simulink model "pd_nf_pi_dvco"  (R2024b)
settings: configuration reference "CONFI" (kept outside this file)
libraries: slpidlib x1
settings Model: DataDictionary=dic_pfc3ph.sldd  Creator=ASUSTUF  LastModifiedBy=Angel
settings ConfigSetRef: SourceName=CONFI

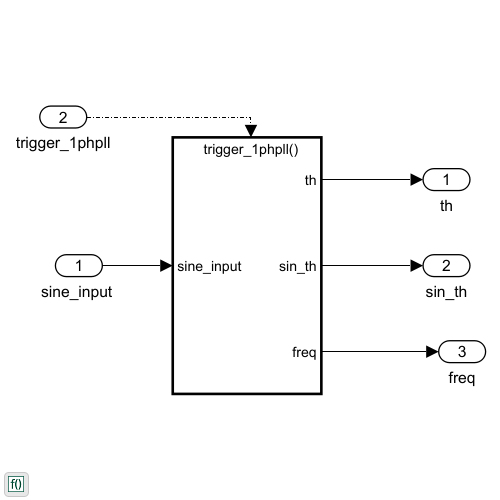
[thumbnail: Simulink's stored preview of the top-level diagram]
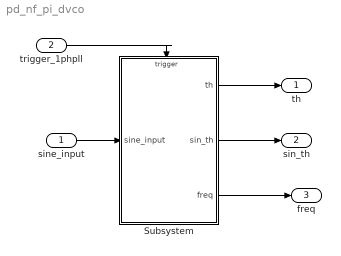
== system pd_nf_pi_dvco ==
  "sine_input " : Inport
  trigger_1phpll : Inport  Port=2  OutputFunctionCall=on
  Subsystem : Subsystem
  th : Outport
  sin_th : Outport  Port=2
  freq : Outport  Port=3
  wires:
  "sine_input "/1 -> Subsystem/1("sine_input ")
  Subsystem/1(th) -> th/1
  Subsystem/2(sin_th) -> sin_th/1
  Subsystem/3(freq) -> freq/1
  trigger_1phpll/1 -> Subsystem/Trigger

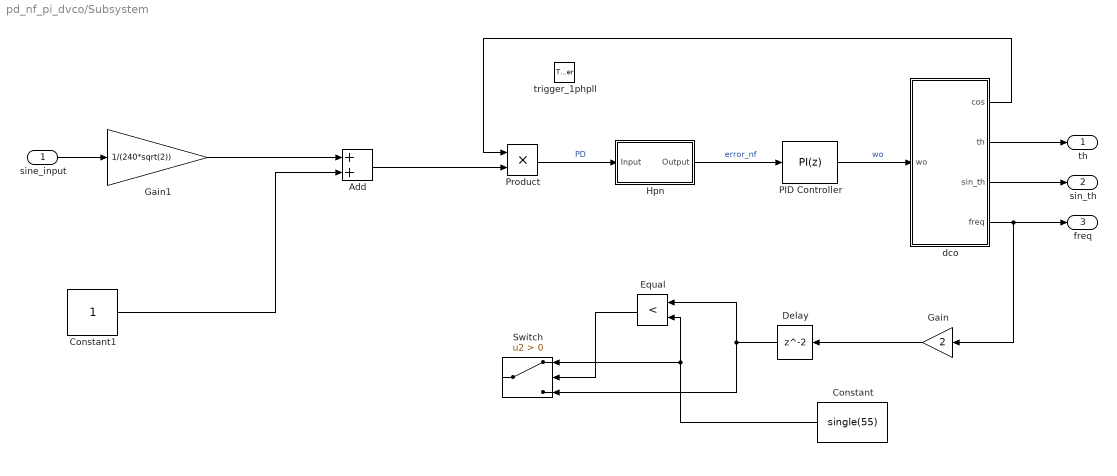
== system pd_nf_pi_dvco/Subsystem ==
  "sine_input " : Inport
  trigger_1phpll : TriggerPort  TriggerType=function-call  VariantControl=(inherit)  PortDimensions=1
  Add : Sum
  Constant : Constant  Value=single(55)  OutDataTypeStr=single  SampleTime=-1
  Constant1 : Constant  OutDataTypeStr=single  SampleTime=-1
  Delay : Delay  InitialCondition=single(2*55)
  Equal : RelationalOperator  Operator=<  OutDataTypeStr=boolean  RndMeth=Simplest  InputSameDT=off
  Gain : Gain  Gain=2  OutDataTypeStr=single
  Gain1 : Gain  Gain=1/(240*sqrt(2))  OutDataTypeStr=single
  Hpn : Subsystem  Tag=FilterWizardSubSystem
      settings: ErrorFcn=dspFilterRealizedInBasicElemsAlgLoopErrFcnCallback
  PID Controller : slpidlib/PID Controller  Controller=PI  Form=Parallel  TimeDomain=Discrete-time  UseExternalTs=on  SampleTime=-1  IntegratorMethod=Forward Euler  FilterMethod=Forward Euler  ControllerParametersSource=internal  P=1  I=.1  UseKiTs=on  D=60  UseExternalDerivativeSource=off  N=5  UseFilter=on  TunerSelectOption=Transfer Function Based (PID Tuner App)  InitialConditionSource=internal  InitialConditionForIntegrator=0  InitialConditionForFilter=0  DifferentiatorICPrevScaledInput=0  ExternalReset=none  TrackingMode=off  Kt=1  LimitOutput=off  SatLimitsSource=internal  UpperSaturationLimit=inf  LowerSaturationLimit=-inf  LinearizeAsGain=on  AntiWindupMode=none  Kb=1  LimitIntegrator=off  UpperIntegratorSaturationLimit=inf  LowerIntegratorSaturationLimit=-inf  PGainOutDataTypeStr=single  PProdOutDataTypeStr=single  POutMin=[]  POutMax=[]  IGainOutDataTypeStr=single  IProdOutDataTypeStr=single  IOutMin=[]  IOutMax=[]  DOutMin=[]  DOutMax=[]  NOutMin=[]  NOutMax=[]  SumOutDataTypeStr=single  SumOutMin=[]  SumOutMax=[]  SaturationOutMin=[]  SaturationOutMax=[]  PParamMin=[]  PParamMax=[]  IParamMin=[]  IParamMax=[]  DParamMin=[]  DParamMax=[]  NParamMin=[]  NParamMax=[]  KbParamMin=[]  KbParamMax=[]  KtParamMin=[]  KtParamMax=[]  KbOutMin=[]  KbOutMax=[]  KtOutMin=[]  KtOutMax=[]  IntegratorOutMin=[]  IntegratorOutMax=[]  FilterOutMin=[]  FilterOutMax=[]  SumI1OutMin=[]  SumI1OutMax=[]  SumI2OutMin=[]  SumI2OutMax=[]  SumI3OutMin=[]  SumI3OutMax=[]  SumI4OutMin=[]  SumI4OutMax=[]  SumDOutMin=[]  SumDOutMax=[]  DifferentiatorOutMin=[]  DifferentiatorOutMax=[]  FilterDiffOutCoefMin=[]  FilterDiffOutCoefMax=[]  ReciprocalOutMin=[]  ReciprocalOutMax=[]  SumDenOutMin=[]  SumDenOutMax=[]  SumNumOutMin=[]  SumNumOutMax=[]  DivideOutMin=[]  DivideOutMax=[]  UdiffTsProdOutMin=[]  UdiffTsProdOutMax=[]  NTsProdOutMin=[]  NTsProdOutMax=[]  UintegralTsProdOutMin=[]  UintegralTsProdOutMax=[]  UngainTsProdOutMin=[]  UngainTsProdOutMax=[]  ClampingZeroOutDataTypeStr=Inherit: Inherit via back propagation  ClampingZeroOutMin=[]  ClampingZeroOutMax=[]  FilterDenConstantOutDataTypeStr=Inherit: Inherit via back propagation  FilterDenConstantOutMin=[]  FilterDenConstantOutMax=[]  PCopyOutDataTypeStr=Inherit: Inherit via back propagation  PCopyOutMin=[]  PCopyOutMax=[]  NCopyOutDataTypeStr=Inherit: Inherit via back propagation  NCopyOutMin=[]  NCopyOutMax=[]  IntegratorContinuousStateAttributes=''  IntegratorStateMustResolveToSignalObject=off  IntegratorRTWStateStorageClass=Auto  FilterContinuousStateAttributes=''  FilterStateMustResolveToSignalObject=off  FilterRTWStateStorageClass=Auto  ParallelPVariant=InternalParameters  IdealPVariant=Disabled  IVariant=InternalParameters  DVariant=Disabled  IntegratorVariant=Discrete  SatVariant=Disabled  AWVariant=Passthrough  PCopyVariant=Disabled  TRVariant=Disabled  FdbkBlocksVariant=Forward  IdealPFdbkVariant=Disabled  SatFdbkVariant=Disabled  DerivativeFilterVariant=Disabled  NVariant=Disabled  NCopyVariant=Disabled_SignalSpec  FilterICVariant=Disabled  IntegratorICVariant=InternalICs  ExternalResetVariant=Disabled  TRSumVariant=Passthrough  SumFdbkVariant=Disabled  SumVariant=Sum_PI  TsampFilterVariant=InternalTs  TsampNgainVariant=Passthrough  TsampIntegralVariant=Passthrough  ExternalSaturationOutDataTypeStr=Inherit: Same as second input  DerivativeSourceVariant=Disabled  PreIntVariant=InternalPreInt
  Product : Product  OutDataTypeStr=single
  Switch : Switch  Criteria=u2 > Threshold  SaturateOnIntegerOverflow=off  InputSameDT=off
  dco : Subsystem
  th : Outport
  sin_th : Outport  Port=2
  freq : Outport  Port=3
  wires:
  dco/1(cos) -> Product/1
  Product/1 -> Hpn/1(Input)  "PD"
  Constant1/1 -> Add/2
  PID Controller/1 -> dco/1(wo)  "wo"
  Equal/1 -> Switch/2
  Gain/1 -> Delay/1
  Hpn/1(Output) -> PID Controller/1  "error_nf"
  dco/3(sin_th) -> sin_th/1
  dco/4(freq) -> freq/1, Gain/1
  "sine_input "/1 -> Gain1/1
  dco/2(th) -> th/1
  Constant/1 -> Switch/1, Equal/2
  Add/1 -> Product/2
  Delay/1 -> Switch/3, Equal/1
  Gain1/1 -> Add/1

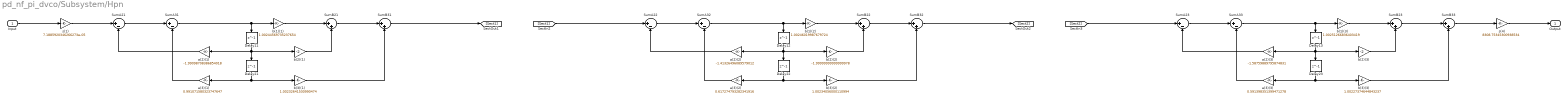
== system pd_nf_pi_dvco/Subsystem/Hpn ==
  Input : Inport
  Delay{11..13,21..23} (6 alike) : Delay  DelayLength=1  InitialCondition=0
  SumA{21..23,31..33} (6 alike) : Sum  Inputs=|+-  RndMeth=Nearest  SaturateOnIntegerOverflow=on  OutDataTypeStr=Inherit: Same as first input
  SumB{21..23,31..33} (6 alike) : Sum  Inputs=|++  RndMeth=Nearest  SaturateOnIntegerOverflow=on  OutDataTypeStr=Inherit: Same as first input
  a(2)(1) : Gain  Gain=-1.99098708386854018  ParamDataTypeStr=single  RndMeth=Nearest  SaturateOnIntegerOverflow=on  OutDataTypeStr=Inherit: Same as input
  a(2)(2) : Gain  Gain=-1.41326496089579012  ParamDataTypeStr=single  RndMeth=Nearest  SaturateOnIntegerOverflow=on  OutDataTypeStr=Inherit: Same as input
  a(2)(3) : Gain  Gain=-1.58759889795874831  ParamDataTypeStr=single  RndMeth=Nearest  SaturateOnIntegerOverflow=on  OutDataTypeStr=Inherit: Same as input
  a(3)(1) : Gain  Gain=0.991071580323747647  ParamDataTypeStr=single  RndMeth=Nearest  SaturateOnIntegerOverflow=on  OutDataTypeStr=Inherit: Same as input
  a(3)(2) : Gain  Gain=0.617274793282341916  ParamDataTypeStr=single  RndMeth=Nearest  SaturateOnIntegerOverflow=on  OutDataTypeStr=Inherit: Same as input
  a(3)(3) : Gain  Gain=0.591398351399471278  ParamDataTypeStr=single  RndMeth=Nearest  SaturateOnIntegerOverflow=on  OutDataTypeStr=Inherit: Same as input
  b(1)(1) : Gain  Gain=1.00244569735237654  ParamDataTypeStr=single  RndMeth=Nearest  SaturateOnIntegerOverflow=on  OutDataTypeStr=Inherit: Same as input
  b(1)(2) : Gain  Gain=1.00246019987679724  ParamDataTypeStr=single  RndMeth=Nearest  SaturateOnIntegerOverflow=on  OutDataTypeStr=Inherit: Same as input
  b(1)(3) : Gain  Gain=1.00251266836403419  ParamDataTypeStr=single  RndMeth=Nearest  SaturateOnIntegerOverflow=on  OutDataTypeStr=Inherit: Same as input
  b(2)(1) : Gain  Gain=-2  ParamDataTypeStr=single  RndMeth=Nearest  SaturateOnIntegerOverflow=on  OutDataTypeStr=Inherit: Same as input
  b(2)(2) : Gain  Gain=-1.99999999999999978  ParamDataTypeStr=single  RndMeth=Nearest  SaturateOnIntegerOverflow=on  OutDataTypeStr=Inherit: Same as input
  b(2)(3) : Gain  Gain=-2  ParamDataTypeStr=single  RndMeth=Nearest  SaturateOnIntegerOverflow=on  OutDataTypeStr=Inherit: Same as input
  b(3)(1) : Gain  Gain=1.00232641530990474  ParamDataTypeStr=single  RndMeth=Nearest  SaturateOnIntegerOverflow=on  OutDataTypeStr=Inherit: Same as input
  b(3)(2) : Gain  Gain=1.00234056000110994  ParamDataTypeStr=single  RndMeth=Nearest  SaturateOnIntegerOverflow=on  OutDataTypeStr=Inherit: Same as input
  b(3)(3) : Gain  Gain=1.00227374644843237  ParamDataTypeStr=single  RndMeth=Nearest  SaturateOnIntegerOverflow=on  OutDataTypeStr=Inherit: Same as input
  s(1) : Gain  Gain=7.1885920346266273e-05  ParamDataTypeStr=single  RndMeth=Nearest  SaturateOnIntegerOverflow=on  OutDataTypeStr=Inherit: Same as input
  s(4) : Gain  Gain=8308.75345300938534  ParamDataTypeStr=single  RndMeth=Nearest  SaturateOnIntegerOverflow=on  OutDataTypeStr=Inherit: Same as input
  Output : Outport
  wires:
  Input/1 -> s(1)/1
  s(1)/1 -> SumA21/1
  SumA21/1 -> SumA31/1
  SumA31/1 -> b(1)(1)/1, Delay11/1
  b(1)(1)/1 -> SumB21/1
  SumB21/1 -> SumB31/1
  SumB31/1 -> [Sect1]
  a(2)(1)/1 -> SumA21/2
  Delay11/1 -> a(2)(1)/1, b(2)(1)/1, Delay21/1
  b(2)(1)/1 -> SumB21/2
  a(3)(1)/1 -> SumA31/2
  Delay21/1 -> a(3)(1)/1, b(3)(1)/1
  b(3)(1)/1 -> SumB31/2
  [Sect1] -> SumA22/1
  SumA22/1 -> SumA32/1
  SumA32/1 -> b(1)(2)/1, Delay12/1
  b(1)(2)/1 -> SumB22/1
  SumB22/1 -> SumB32/1
  SumB32/1 -> [Sect2]
  a(2)(2)/1 -> SumA22/2
  Delay12/1 -> a(2)(2)/1, b(2)(2)/1, Delay22/1
  b(2)(2)/1 -> SumB22/2
  a(3)(2)/1 -> SumA32/2
  Delay22/1 -> a(3)(2)/1, b(3)(2)/1
  b(3)(2)/1 -> SumB32/2
  [Sect2] -> SumA23/1
  SumA23/1 -> SumA33/1
  SumA33/1 -> b(1)(3)/1, Delay13/1
  b(1)(3)/1 -> SumB23/1
  SumB23/1 -> SumB33/1
  SumB33/1 -> s(4)/1
  a(2)(3)/1 -> SumA23/2
  Delay13/1 -> a(2)(3)/1, b(2)(3)/1, Delay23/1
  b(2)(3)/1 -> SumB23/2
  a(3)(3)/1 -> SumA33/2
  Delay23/1 -> a(3)(3)/1, b(3)(3)/1
  b(3)(3)/1 -> SumB33/2
  s(4)/1 -> Output/1

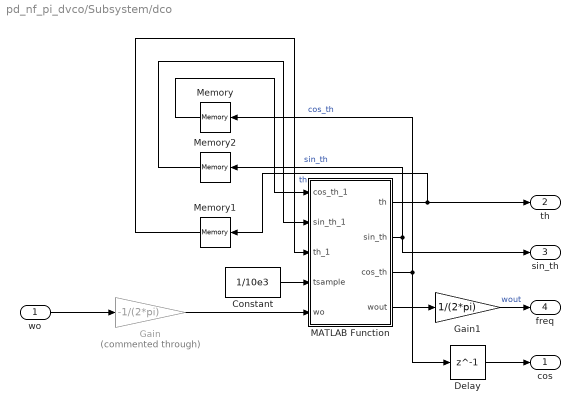
== system pd_nf_pi_dvco/Subsystem/dco ==
  wo : Inport
  Constant : Constant  Value=1/10e3  OutDataTypeStr=single  SampleTime=-1
  Delay : Delay  DelayLength=1  InitialCondition=single(0')
  Gain : Gain  Commented=through  Gain=-1/(2*pi)
  Gain1 : Gain  Gain=1/(2*pi)  OutDataTypeStr=single
  MATLAB Function : MATLAB Function  TreatAsAtomicUnit=on
  Memory : Memory  InitialCondition=.99  InheritSampleTime=on
  Memory1 : Memory  InheritSampleTime=on
  Memory2 : Memory  InheritSampleTime=on
  cos : Outport
  th : Outport  Port=2
  sin_th : Outport  Port=3
  freq : Outport  Port=4
  wires:
  wo/1 -> Gain/1
  Constant/1 -> MATLAB Function/4(tsample)
  Memory1/1 -> MATLAB Function/3(th_1)
  Memory2/1 -> MATLAB Function/2(sin_th_1)
  Memory/1 -> MATLAB Function/1(cos_th_1)
  Delay/1 -> cos/1
  MATLAB Function/1(th) -> Memory1/1, th/1  "th"
  MATLAB Function/2(sin_th) -> sin_th/1, Memory2/1  "sin_th"
  MATLAB Function/3(cos_th) -> Delay/1, Memory/1  "cos_th"
  Gain/1 -> MATLAB Function/5(wo)
  MATLAB Function/4(wout) -> Gain1/1
  Gain1/1 -> freq/1  "wout"

== matlab function pd_nf_pi_dvco/Subsystem/dco/MATLAB Function ==
  data: cos_th_1 input; sin_th_1 input; th_1 input; tsample input; th output; sin_th output; wo input; cos_th output; wout output
 function [th,sin_th,cos_th,wout]= dco(cos_th_1,sin_th_1,th_1,tsample,wo)
        ws=single(2*pi*50);
        wout=single(wo+ws);
        
        %Sin is for showing the overlaping w the input 
        sin_th=sin_th_1+(cos_th_1*wout*tsample);%Sin(t+dt)=sin(t)+cos(t)*dt
        cos_th=cos_th_1-(sin_th_1*wout*tsample);
        
        sin_th=max([sin_th -1]);
        cos_th=max([cos_th -1]);

        sin_th=min([sin_th 1]);
        cos_th=min([cos_th 1]);

        th=th_1+(wout*tsample);

         if sin_th>=0 && sin_th_1<=0
            th=single(0);    %fi(pi,1,32,29); %zero crossing reseting phase angle
        end
      
end
